simulink model "ADC_DFT"  (R2013a)
settings: Solver=ode45  StartTime=0.0  StopTime=90  RelTol=1e-3
PostLoadFcn:
  | bps_model_init(gcs);
undefined symbols (not defined in the file): xlipgetpartsetting
libraries: xbsIndex_r4 x73, xps_library x22, mbee4_library x4
(part 1 of 3)
settings Model: Creator=BEEcube  LastModifiedBy=rijesh
settings DataIOCC: SignalLoggingSaveFormat=ModelDataLogs
settings OptimizationCC: InlineParams=on  ExpressionDepthLimit=2147483647
settings DebuggingCC: FcnCallInpInsideContextMsg=UseLocalSettings
settings GRTTargetCC: CombineOutputUpdateFcns=off  GRTInterface=on

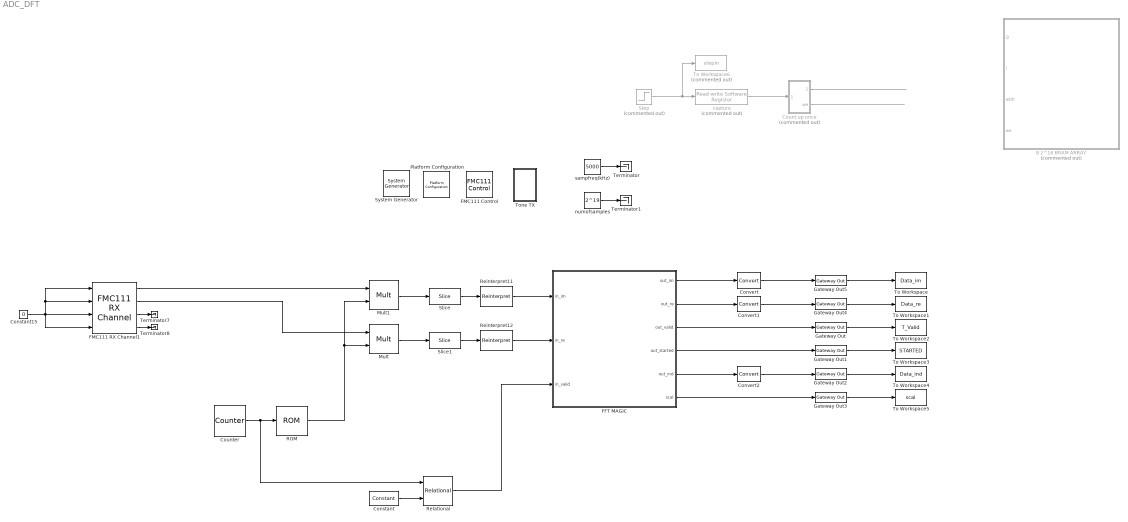
== system ADC_DFT ==
  " Platform Configuration " : mbee4_library/ Platform Configuration   Tag=xps:xsg,ver:4.5  xsg_ver=14.7  hw_sys=mBEE4  fpga_type=xc6vsx475t  fpga_device='xc6vsx475t-2ff1759'  bp_override=off  bp_choice='mBEE4'  bp_option=base  clk_src=fmc_clk1_fx: User defined clock based on FMC_HPC_CLK1  clk_rate=250000000  ref_clk_rate=250000000  enable_half_rate=off  sample_period=1  update=off
  " System Generator" : xbsIndex_r4/ System Generator  Tag=genX  xilinxfamily=virtex6  part=xc6vsx475t  speed=-2  package=ff1759  synthesis_tool=XST  clock_wrapper=Clock Enables  directory=./radarDFT/sysgen  proj_type=Project Navigator  Synth_file=XST Defaults  Impl_file=ISE Defaults  testbench=off  simulink_period=1  sysclk_period=4  dcm_input_clock_period=10  incr_netlist=off  trim_vbits=Everywhere in SubSystem  dbl_ovrd=According to Block Masks  core_generation=According to Block Masks  run_coregen=off  deprecated_control=off  eval_field=0  block_type=sysgen
  8 2^16 BRAM ARRAY : Subsystem  Commented=on
  Constant : xbsIndex_r4/Constant  const=252  gui_display_data_type=Fixed-point  arith_type=Unsigned  n_bits=8  bin_pt=0  preci_type=Single  exp_width=8  frac_width=24  explicit_period=off  period=1  equ=P=C  opselect=C  inp2=PCIN>>17  opr=+  inp1=P  carry=CIN  dbl_ovrd=off  block_type=constant
  Constant15 : Constant  Value=0  SampleTime=1
  Convert : xbsIndex_r4/Convert  gui_display_data_type=Fixed-point  arith_type="Signed  (2's comp)"  n_bits=14  bin_pt=0  float_type=Double  exp_bits=8  fraction_bits=24  quantization=Truncate  overflow=Wrap  en=off  latency=0  dbl_ovrd=off  pipeline=off  block_type=convert
  Convert1 : xbsIndex_r4/Convert  gui_display_data_type=Fixed-point  arith_type="Signed  (2's comp)"  n_bits=14  bin_pt=0  float_type=Double  exp_bits=8  fraction_bits=24  quantization=Truncate  overflow=Wrap  en=off  latency=0  dbl_ovrd=off  pipeline=off  block_type=convert
  Convert2 : xbsIndex_r4/Convert  gui_display_data_type=Fixed-point  arith_type=Unsigned  n_bits=8  bin_pt=0  float_type=Double  exp_bits=8  fraction_bits=24  quantization=Truncate  overflow=Wrap  en=off  latency=0  dbl_ovrd=off  pipeline=off  block_type=convert
  Count up once : Subsystem  Commented=on
  Counter : xbsIndex_r4/Counter  cnt_type=Free Running  cnt_to=Inf  operation=Up  start_count=0  cnt_by_val=1  arith_type=Unsigned  n_bits=8  bin_pt=0  load_pin=off  rst=off  en=off  explicit_period=on  period=1  dbl_ovrd=off  use_behavioral_HDL=off  implementation=Fabric  block_type=counter
  FFT MAGIC : Subsystem
  FMC111 Control : mbee4_library/FMC111 Control  Tag=xps:fmc111_ctrl  board_type=FMC111  sample_period=1  update=off
  FMC111 RX Channel1 : mbee4_library/FMC111 RX Channel  Tag=xps:fmc111_rx  channel_number=1  arith_type=Signed  bitwidth=14  bin_pt=0  sample_period=1  update=off
  Gateway Out{,1..5} (6 alike) : xbsIndex_r4/Gateway Out  inherit_from_input=off  hdl_port=on  timing_constraint=None  locs_specified=off  LOCs={}  UseAsDAC=off  DACChannel='1'  block_type=gatewayout
  Mult : xbsIndex_r4/Mult  precision=Full  arith_type="Signed  (2's comp)"  n_bits=16  bin_pt=14  quantization=Truncate  overflow=Wrap  en=off  latency=3  dbl_ovrd=off  use_behavioral_HDL=off  opt=Speed  use_embedded=on  optimum_pipeline=off  pipeline=on  use_rpm=on  placement_style=Triangular  block_type=mult
  Mult1 : xbsIndex_r4/Mult  precision=Full  arith_type="Signed  (2's comp)"  n_bits=16  bin_pt=14  quantization=Truncate  overflow=Wrap  en=off  latency=3  dbl_ovrd=off  use_behavioral_HDL=off  opt=Speed  use_embedded=on  optimum_pipeline=off  pipeline=on  use_rpm=on  placement_style=Triangular  block_type=mult
  ROM : xbsIndex_r4/ROM  depth=256  initVector=0.5*(1-cos(2*pi*(0:255)/255))  distributed_mem=Distributed memory  rst=off  init_reg=0  en=off  latency=1  gui_display_data_type=Fixed-point  arith_type="Signed  (2's comp)"  n_bits=16  bin_pt=14  preci_type=Single  exp_width=8  frac_width=24  dbl_ovrd=off  optimize=Area  use_rpm=on  block_type=sprom
  Reinterpret11 : xbsIndex_r4/Reinterpret  force_arith_type=on  arith_type="Signed  (2's comp)"  force_bin_pt=on  bin_pt=13  block_type=reinterpret
  Reinterpret12 : xbsIndex_r4/Reinterpret  force_arith_type=on  arith_type="Signed  (2's comp)"  force_bin_pt=on  bin_pt=13  block_type=reinterpret
  Relational : xbsIndex_r4/Relational  mode=a=b  en=off  latency=0  dbl_ovrd=off  block_type=relational
  Slice : xbsIndex_r4/Slice  nbits=14  boolean_output=off  mode=Lower Bit Location + Width  bit1=0  base1=MSB of Input  bit0=14  base0=LSB of Input  dbl_ovrd=off  block_type=slice
  Slice1 : xbsIndex_r4/Slice  nbits=14  boolean_output=off  mode=Lower Bit Location + Width  bit1=0  base1=MSB of Input  bit0=14  base0=LSB of Input  dbl_ovrd=off  block_type=slice
  Step : Step  Commented=on  SampleTime=1
  Terminator{,1,7..8} (4 alike) : Terminator
  To Workspace : ToWorkspace  VariableName=Data_im  SampleTime=-1  SaveFormat=Timeseries
  To Workspace1 : ToWorkspace  VariableName=Data_re  SampleTime=-1  SaveFormat=Timeseries
  To Workspace2 : ToWorkspace  VariableName=T_Valid  SampleTime=-1  SaveFormat=Timeseries
  To Workspace3 : ToWorkspace  VariableName=STARTED  SampleTime=-1  SaveFormat=Timeseries
  To Workspace4 : ToWorkspace  VariableName=Data_ind  SampleTime=-1  SaveFormat=Timeseries
  To Workspace5 : ToWorkspace  VariableName=scal  SampleTime=-1  SaveFormat=Timeseries
  To Workspace6 : ToWorkspace  Commented=on  VariableName=stepin  SampleTime=-1
  Tone TX : Subsystem  VariantControl=Variant1
  capture : xps_library/Read-write Software Register  Tag=xps:sw_reg  Commented=on  io_dir=From Processor  use_strobe=off  arith_type=Unsigned  bitwidth=32  bin_pt=0  sample_period=1  update=off
  numofsamples : Constant  Value=2^19
  sampfreq(kHz) : Constant  Value=5000
  wires:
  Step/1 -> capture/1, To Workspace6/1
  Constant15/1 -> FMC111 RX Channel1/4, FMC111 RX Channel1/3, FMC111 RX Channel1/2, FMC111 RX Channel1/1
  FMC111 RX Channel1/3 -> Terminator7/1
  FMC111 RX Channel1/4 -> Terminator8/1
  Mult1/1 -> Slice/1
  FMC111 RX Channel1/2 -> Mult/1
  sampfreq(kHz)/1 -> Terminator/1
  numofsamples/1 -> Terminator1/1
  capture/1 -> Count up once/1(start)
  Count up once/1(addr) -> ?
  Count up once/2(we) -> ?
  Relational/1 -> FFT MAGIC/3(in_valid)
  FFT MAGIC/5(out_ind) -> Convert2/1
  FFT MAGIC/4(out_started) -> Gateway Out1/1
  FFT MAGIC/3(out_valid) -> Gateway Out/1
  FFT MAGIC/1(out_im) -> Convert/1
  FFT MAGIC/2(out_re) -> Convert1/1
  Gateway Out5/1 -> To Workspace/1
  Gateway Out4/1 -> To Workspace1/1
  Gateway Out/1 -> To Workspace2/1
  Gateway Out1/1 -> To Workspace3/1
  Gateway Out2/1 -> To Workspace4/1
  Convert1/1 -> Gateway Out4/1
  Convert/1 -> Gateway Out5/1
  Convert2/1 -> Gateway Out2/1
  FFT MAGIC/6(scal) -> Gateway Out3/1
  Gateway Out3/1 -> To Workspace5/1
  ROM/1 -> Mult1/2, Mult/2
  Mult/1 -> Slice1/1
  Counter/1 -> Relational/1, ROM/1
  FMC111 RX Channel1/1 -> Mult1/1
  Reinterpret11/1 -> FFT MAGIC/1(in_im)
  Reinterpret12/1 -> FFT MAGIC/2(in_re)
  Slice/1 -> Reinterpret11/1
  Slice1/1 -> Reinterpret12/1
  Constant/1 -> Relational/2
